simulink model "Spindel_Test"  (Simulink 7.7)
settings: Solver=ode45  StartTime=0.0  StopTime=20  RelTol=1e-3
libraries: WZM_QSS_Lib x1
settings Model: Creator=simon  LastModifiedBy=Coni

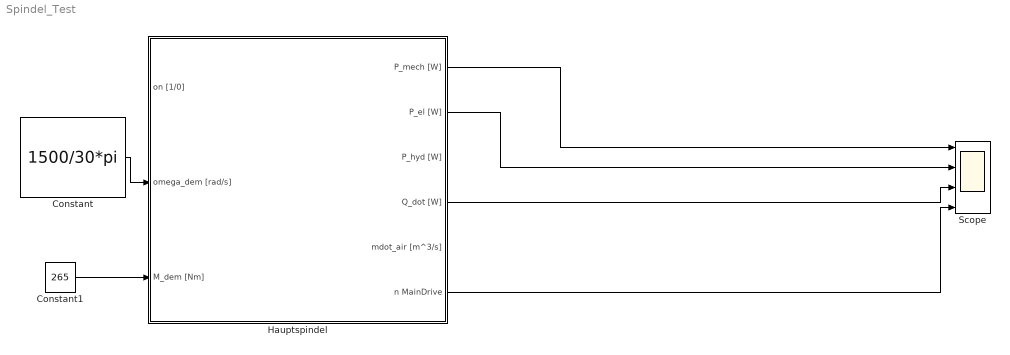
== system Spindel_Test ==
  Constant : Constant  Value=1500/30*pi
  Constant1 : Constant  Value=265
  Hauptspindel : Subsystem  BlockChoice=MainDrive_simple
      link override MainDrive_simple: P_max=40e3
      settings: TemplateBlock=WZM_QSS_Lib/Drives/MainDrive  MemberBlocks=MainDrive_Dummy,MainDrive_simple
  Scope : Scope  NumInputPorts=4
      settings: TimeRange=20  YMin=0~0~0~0  YMax=50000~300000~300000~0.8
  wires:
  Hauptspindel/1(P_mech [W]) -> Scope/1
  Hauptspindel/2(P_el [W]) -> Scope/2
  Hauptspindel/4(Q_dot [W]) -> Scope/3
  Hauptspindel/6(n MainDrive) -> Scope/4
  Constant/1 -> Hauptspindel/2(omega_dem [rad/s])
  Constant1/1 -> Hauptspindel/3(M_dem [Nm])

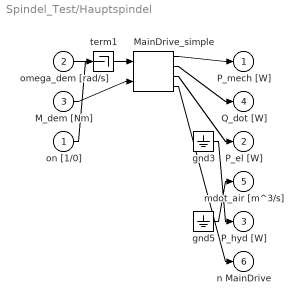
== system Spindel_Test/Hauptspindel ==
  on [1/0] : Inport
  omega_dem [rad/s] : Inport  Port=2
  M_dem [Nm] : Inport  Port=3
  MainDrive_simple : WZM_QSS_Lib/Drives/MainDrive_simple  SystemSampleTime=-1  P_max=40e3  eta=0.92  theta=1  Tomega=MainDrive.Tabelomega  TM=MainDrive.TabelM  Teta=MainDrive.Tabeleta
  gnd3 : Ground
  gnd5 : Ground
  term1 : Terminator
  P_mech [W] : Outport
  P_el [W] : Outport  Port=2
  P_hyd [W] : Outport  Port=3
  Q_dot [W] : Outport  Port=4
  mdot_air [m^3/s] : Outport  Port=5
  n MainDrive : Outport  Port=6
  wires:
  omega_dem [rad/s]/1 -> MainDrive_simple/1
  M_dem [Nm]/1 -> MainDrive_simple/2
  MainDrive_simple/1 -> P_mech [W]/1
  MainDrive_simple/2 -> Q_dot [W]/1
  MainDrive_simple/3 -> P_el [W]/1
  MainDrive_simple/4 -> n MainDrive/1
  on [1/0]/1 -> term1/1
  gnd3/1 -> P_hyd [W]/1
  gnd5/1 -> mdot_air [m^3/s]/1
